simulink model "robott10"  (R2018b)
settings: Solver=VariableStepAuto  StartTime=0.0  StopTime=5  RelTol=1e-3
settings Model: Creator=User  LastModifiedBy=User

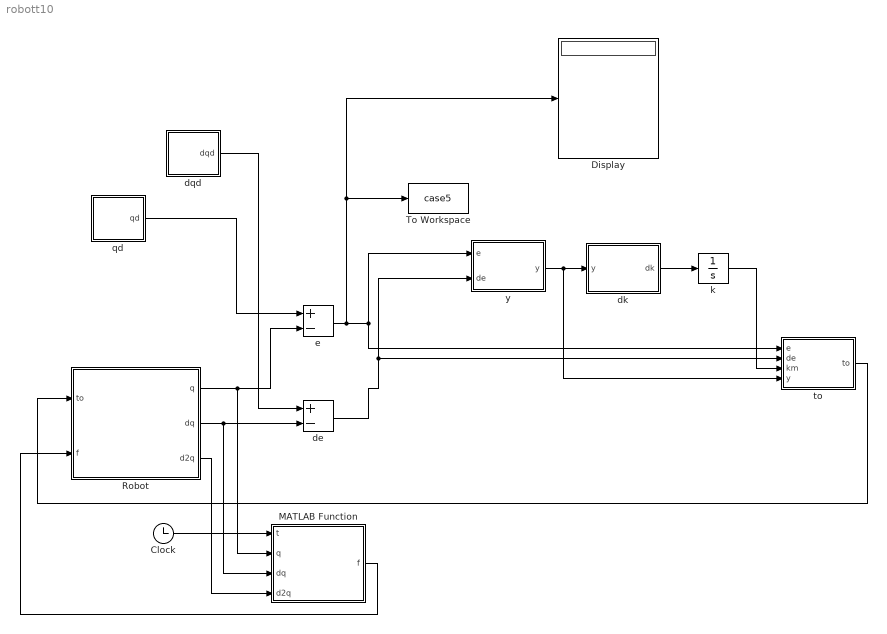
== system robott10 ==
  Clock : Clock
  Display : Display
  MATLAB Function : MATLAB Function  TreatAsAtomicUnit=on
  Robot : Subsystem
  To Workspace : ToWorkspace  VariableName=case5  SaveFormat=Timeseries  SampleTime=-1
  de : Sum  Inputs=+-
  dk : MATLAB Function  TreatAsAtomicUnit=on
  dqd : Subsystem
  e : Sum  Inputs=+-
  k : Integrator  InitialCondition=[0;0;0;0;0;0]
  qd : Subsystem
  to : MATLAB Function  TreatAsAtomicUnit=on
  y : MATLAB Function  TreatAsAtomicUnit=on
  wires:
  MATLAB Function/1(f) -> Robot/2(f)
  qd/1(qd) -> e/1
  Robot/1(q) -> MATLAB Function/2(q), e/2
  Robot/2(dq) -> MATLAB Function/3(dq), de/2
  dqd/1(dqd) -> de/1
  e/1 -> y/1(e), to/1(e), To Workspace/1, Display/1
  de/1 -> y/2(de), to/2(de)
  to/1(to) -> Robot/1(to)
  y/1(y) -> to/4(y), dk/1(y)
  dk/1(dk) -> k/1
  k/1 -> to/3(km)
  Clock/1 -> MATLAB Function/1(t)
  Robot/3(d2q) -> MATLAB Function/4(d2q)

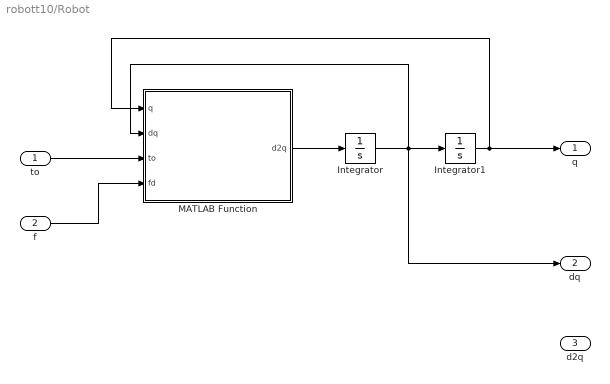
== system robott10/Robot ==
  to : Inport
  f : Inport  Port=2
  Integrator : Integrator  InitialCondition=[0;0;0;0;0;0]
  Integrator1 : Integrator  InitialCondition=[0;0;0;0;0;0]
  MATLAB Function : MATLAB Function  TreatAsAtomicUnit=on
  q : Outport
  dq : Outport  Port=2
  d2q : Outport  Port=3
  wires:
  MATLAB Function/1(d2q) -> Integrator/1
  Integrator/1 -> dq/1, MATLAB Function/2(dq), Integrator1/1
  Integrator1/1 -> q/1, MATLAB Function/1(q)
  to/1 -> MATLAB Function/3(to)
  f/1 -> MATLAB Function/4(fd)

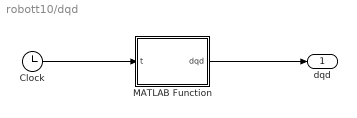
== system robott10/dqd ==
  Clock : Clock
  MATLAB Function : MATLAB Function  TreatAsAtomicUnit=on
  dqd : Outport
  wires:
  MATLAB Function/1(dqd) -> dqd/1
  Clock/1 -> MATLAB Function/1(t)

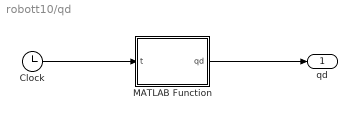
== system robott10/qd ==
  Clock : Clock
  MATLAB Function : MATLAB Function  TreatAsAtomicUnit=on
  qd : Outport
  wires:
  Clock/1 -> MATLAB Function/1(t)
  MATLAB Function/1(qd) -> qd/1

== matlab function robott10/qd/MATLAB Function ==
  data: t input; qd output
function qd = fcn(t)
qd=(12*(t/5)^5-30*(t/5)^4+20*(t/5)^3)*ones(6,1);
end

== matlab function robott10/Robot/MATLAB Function ==
  data: q input; d2q output; dq input; to input; fd input
function d2q=momenluc(q,dq,to,fd)
d1=0.1397;
a2=0.4318;
d3=0.4337;
d5=0.05588;
q1=q(1);
q2=q(2);
q3=q(3);
q4=q(4);
q5=q(5);
q6=q(6);
A1=[cos(q1) 0 sin(q1) d1*-sin(q1);
    sin(q1) 0 -cos(q1) d1*cos(q1);
    0 1 0 0;
    0 0 0 1];
A2=[cos(q2) -sin(q2) 0 a2*cos(q2);
    sin(q2) cos(q2) 0 a2*sin(q2);
    0 0 1 0;
    0 0 0 1];
A3=[cos(q3) 0 -sin(q3) d3*-sin(q3);
    sin(q3) 0 cos(q3) d3*cos(q3);
    0 -1 0 0;
    0 0 0 1];
A4=[cos(q4) 0 sin(q4) 0;
    sin(q4) 0 -cos(q4) 0;
    0 1 0 0;
    0 0 0 1];
A5=[cos(q5) 0 -sin(q5) -d5*sin(q5);
    sin(q5) 0 cos(q5) d5*cos(q5);
    0 -1 0 0;
    0 0 0 1];
A6=[cos(q6) -sin(q6) 0 0;
    sin(q6) cos(q6) 0 0;
    0 0 1 0;
    0 0 0 1];
A=zeros(4,4,6);
A(:,:,1)=A1;
A(:,:,2)=A2;
A(:,:,3)=A3;
A(:,:,4)=A4;
A(:,:,5)=A5;
A(:,:,6)=A6;
m1=17.4;
m2=4.8;
m3=0.82;
m4=0.34;
m5=0.09;
m6=0.05;
J=zeros(4,4,6);
J(:,:,1)=[0 0 0 0;
    0 0 0 0;
    0 0 m1*d1^2/3 m1*d1/2;
    0 0 m1*d1/2 m1];
J(:,:,2)=[m2*a2^2/3 0 0 -m2*a2/2;
    0 0 0 0;
    0 0 0 0;
    -m2*a2/2 0 0 m2];
J(:,:,3)=[0 0 0 0;
    0 0 0 0;
    0 0 m3*d3^2/3 -m3*d3/2;
    0 0 -m3*d3/2 m3];
J(:,:,4)=[m4*d5^2/4 0 0 0;
    0 m4*d5^2/4 0 0;
    0 0 0 0;
    0 0 0 m4];
J(:,:,5)=[m5*d5^2/4 0 0 0;
    0 0 0 0;
    0 0 5*m5*d5^2/4 -m5*d5;
    0 0 -m5*d5 m5];

J(:,:,6)=[m6*0.05^2 0 0 m6*0.05;
    0 0 0 0;
    0 0 0 0;
    m6*0.05 0 0 m6];
U=zeros(4,4,6,6);
g=[0 0 -9.81 1]';
r=[0 -a2/2 0 0 0 0.05;
    0 0 0 0 0 0;
    d1/2 0 -d3/2 0 -d5 0;
    1 1 1 1 1 1];
for i=1:6
    for j=1:i
        U(:,:,i,j)=eye(4);
        for k=1:j-1
            U(:,:,i,j)=U(:,:,i,j)*A(:,:,k);
        end
        U(:,:,i,j)=U(:,:,i,j)*[0 -1 0 0;1 0 0 0;0 0 0 0;0 0 0 0];
        for k=j:i
            U(:,:,i,j)=U(:,:,i,j)*A(:,:,k);
        end
    end
end
M=zeros(6);
for i=1:6
    for j=i:6
        for k=max(i,j):6
            M(i,j)=M(i,j)+trace(U(:,:,k,j)*J(:,:,k)*U(:,:,k,i)');
        end
        M(j,i)=M(i,j);
    end
end
G=zeros(6,1);
m=[m1;m2;m3;m4;m5;m6];
for i=1:6
    for j=i:6
        G(i)=G(i)+(-m(j)*g'*U(:,:,j,i)*r(:,i));
    end
end
U1=zeros(4,4,6,6,6);
for i=1:6
    for j=1:i
        for k=1:j
            U1(:,:,i,j,k)=eye(4);
            for k1=1:k-1
                U1(:,:,i,j,k)=U1(:,:,i,j,k)*A(:,:,i);
            end
            U1(:,:,i,j,k)=U1(:,:,i,j,k)*[0 -1 0 0;1 0 0 0;0 0 0 0;0 0 0 0];
            for k1=k:j-1
                U1(:,:,i,j,k)=U1(:,:,i,j,k)*A(:,:,i);
            end
            U1(:,:,i,j,k)=U1(:,:,i,j,k)*[0 -1 0 0;1 0 0 0;0 0 0 0;0 0 0 0];
            for k1=j:i
                U1(:,:,i,j,k)=U1(:,:,i,j,k)*A(:,:,i);
            end
            U1(:,:,i,k,j)=U1(:,:,i,j,k);
        end
    end
end
h=zeros(6,6,6);
for i=1:6
    for j=1:6
        for k=1:6
            for k1=max([i,j,k]):6
                h(j,k,i)=h(j,k,i)+trace(U1(:,:,k1,j,k)*J(k1)*U(:,:,k1,i));
            end
        end
    end
end
V=zeros(6,1);
for i=1:6
    V(i)=dq'*h(:,:,i)*dq;
end
d2q=M\(to-V-G-fd);

== matlab function robott10/dqd/MATLAB Function ==
  data: t input; dqd output
function dqd = fcn(t)
dqd=(60*(t/5)^4-120*(t/5)^3+60*(t/5)^2)*1/5*ones(6,1);
end

== matlab function robott10/to ==
  data: e input; to output; de input; km input; y input
function to = fcn(e,de,km,y)
Kp=diag([500 50 50 5 5 5])*2;
Kv=diag([25 5 5 0.5 0.5 0.5])*2;
ve=zeros(6,1);
for i=1:6
if e(i)>=pi/2
    ve(i)=1;
elseif e(i)>-pi/2
    ve(i)=sin(e(i));
else
    ve(i)=-1;
end
end
ye=zeros(6,1);
for i=1:6
if y(i)>=pi/2
    ye(i)=1;
elseif y(i)>-pi/2
    ye(i)=sin(y(i));
else
    ye(i)=-1;
end
end
to=Kp*ve+Kv*de-diag(km)*ye;
end

== matlab function robott10/y ==
  data: e input; y output; de input
function y = fcn(e,de)
muy=1;
ve=zeros(6,1);
for i=1:6
if e(i)>=pi/2
    ve(i)=1;
elseif e(i)>-pi/2
    ve(i)=sin(e(i));
else
    ve(i)=-1;
end
end
y=-de-muy*ve;
end

== matlab function robott10/dk ==
  data: y input; dk output
function dk = fcn(y)
S=diag([1 0.1 0.2 1 1 1])/5;
y_=y.*sign(y);
dk=S\y_;
end

== matlab function robott10/MATLAB Function ==
  data: t input; f output; q input; dq input; d2q input
function f = fcn(t,q,dq,d2q)
ME=0.01*(sin(pi*t))^2;
CE=0.1*(sin(pi*t))^2;
GE=20*(sin(pi*t))^2;
f=ME*d2q+CE*dq+GE*q;
end
